simulink subsystem "request_buffer"  (R2021b)
settings: Solver=VariableStepAuto  StartTime=0.0  StopTime=10.0  RelTol=1e-3
undefined symbols (not defined in the file): id_bitwidth, req_mem_size, ts_bitwidth
libraries: hdlsllib x8, simulink x1
settings Model: Creator=torha  LastModifiedBy=torha
settings SolverCC: AlgebraicLoopSolver=TrustRegion
settings DebuggingCC: SFMachineParentedDataDiag=warning

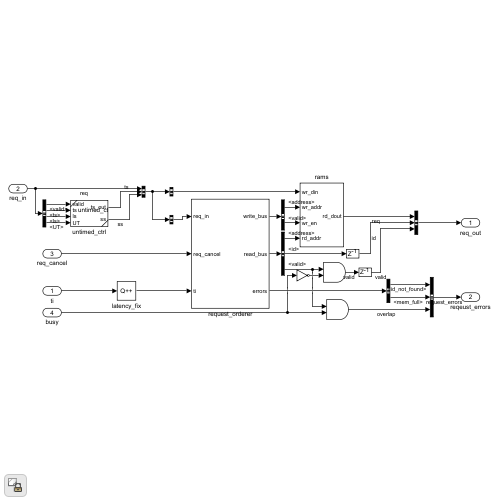
[thumbnail: Simulink's stored preview of the top-level diagram]
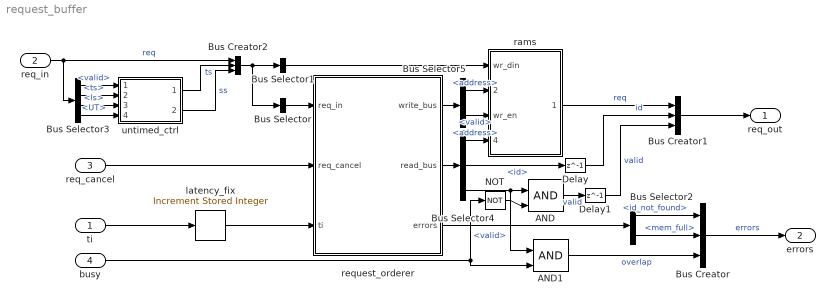
== system request_buffer ==
  ti : Inport
  req_in : Inport  Port=2
  req_cancel : Inport  Port=3
  busy : Inport  Port=4
  AND : Logic  IconShape=distinctive  AllPortsSameDT=off  OutDataTypeStr=boolean
  AND1 : Logic  IconShape=distinctive  AllPortsSameDT=off  OutDataTypeStr=boolean
  Bus Creator : BusCreator  Inputs=3
  Bus Creator1 : BusCreator  Inputs=3
  Bus Creator2 : BusCreator  Inputs=3
  Bus Selector : BusSelector  OutputSignals=req.id,req.valid,ts  OutputAsBus=on
  Bus Selector1 : BusSelector  OutputSignals=req.UC,req.SEND,req.fn,req.filter_address,req.dist_address,ss  OutputAsBus=on
  Bus Selector2 : BusSelector  OutputSignals=signal2.id_not_found,signal2.mem_full
  Bus Selector3 : BusSelector  OutputSignals=valid,ts,ls,UT
  Bus Selector4 : BusSelector  OutputSignals=address,id,valid
  Bus Selector5 : BusSelector  OutputSignals=address,valid
  Delay : Delay  DelayLength=1
  Delay1 : Delay  DelayLength=1
  NOT : Logic  Operator=NOT  IconShape=distinctive  AllPortsSameDT=off  OutDataTypeStr=boolean
  latency_fix : simulink/Additional Math & Discrete/Additional Math: Increment - Decrement/Increment Stored Integer
  rams : Subsystem
  request_orderer : Subsystem
  untimed_ctrl : Subsystem  ReferencedSubsystem=untimed_ctrl
  req_out : Outport
  errors : Outport  Port=2
  wires:
  Bus Selector/1 -> request_orderer/1(req_in)
  busy/1 -> AND1/2, NOT/1
  Bus Creator/1 -> errors/1  "errors"
  AND1/1 -> Bus Creator/3  "overlap"
  req_in/1 -> Bus Creator2/1, Bus Selector3/1  "req"
  NOT/1 -> AND/2
  Bus Selector1/1 -> rams/1(wr_din)
  req_cancel/1 -> request_orderer/2(req_cancel)
  rams/1(rd_dout) -> Bus Creator1/1  "req"
  Bus Selector2/2 -> Bus Creator/2  "<mem_full>"
  Bus Selector2/1 -> Bus Creator/1  "<id_not_found>"
  Bus Creator1/1 -> req_out/1
  Delay/1 -> Bus Creator1/2  "id"
  AND/1 -> Delay1/1  "valid"
  untimed_ctrl/1 -> Bus Creator2/2  "ts"
  Bus Creator2/1 -> Bus Selector1/1, Bus Selector/1
  Bus Selector3/3 -> untimed_ctrl/3  "<ls>"
  Bus Selector3/2 -> untimed_ctrl/2  "<ts>"
  Bus Selector3/4 -> untimed_ctrl/4  "<UT>"
  Bus Selector3/1 -> untimed_ctrl/1  "<valid>"
  untimed_ctrl/2 -> Bus Creator2/3  "ss"
  ti/1 -> latency_fix/1
  Delay1/1 -> Bus Creator1/3  "valid"
  latency_fix/1 -> request_orderer/3(ti)
  request_orderer/3(errors) -> Bus Selector2/1
  request_orderer/2(read_bus) -> Bus Selector4/1
  Bus Selector4/1 -> rams/4(rd_addr)  "<address>"
  Bus Selector5/1 -> rams/2(wr_addr)  "<address>"
  request_orderer/1(write_bus) -> Bus Selector5/1
  Bus Selector5/2 -> rams/3(wr_en)  "<valid>"
  Bus Selector4/3 -> AND/1, AND1/1  "<valid>"
  Bus Selector4/2 -> Delay/1  "<id>"

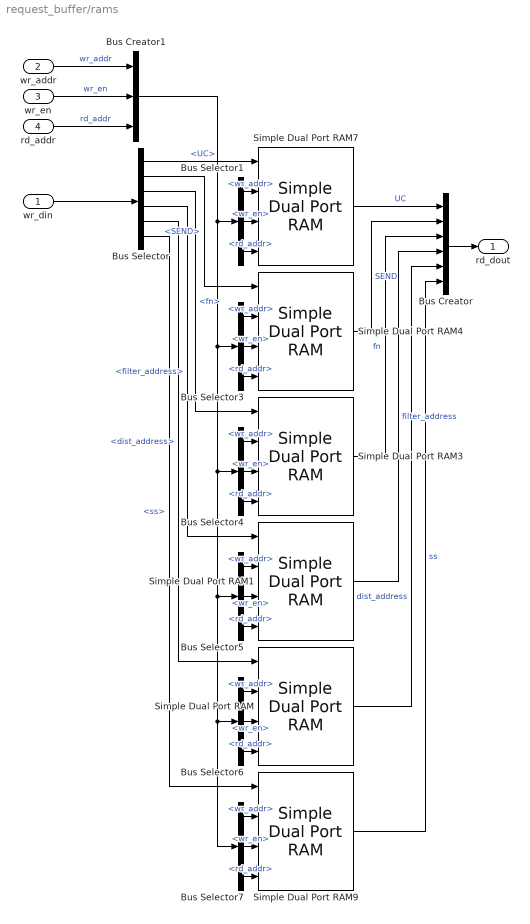
== system request_buffer/rams ==
  wr_din : Inport
  wr_addr : Inport  Port=2
  wr_en : Inport  Port=3
  rd_addr : Inport  Port=4
  Bus Creator : BusCreator  Inputs=6
  Bus Creator1 : BusCreator  Inputs=3
  Bus Selector : BusSelector  OutputSignals=UC,SEND,fn,filter_address,dist_address,ss
  Bus Selector{1,3..7} (6 alike) : BusSelector  OutputSignals=wr_addr,wr_en,rd_addr
  Simple Dual Port RAM{,1,3..4,7,9} (6 alike) : hdlsllib/HDL RAMs/Simple Dual Port RAM  ram_size=log2(req_mem_size)
      settings: SourceProductBaseCode=SL
  rd_dout : Outport
  wires:
  Bus Selector5/3 -> Simple Dual Port RAM1/4  "<rd_addr>"
  Bus Selector5/2 -> Simple Dual Port RAM1/3  "<wr_en>"
  Bus Selector5/1 -> Simple Dual Port RAM1/2  "<wr_addr>"
  Bus Selector4/3 -> Simple Dual Port RAM3/4  "<rd_addr>"
  Bus Selector4/2 -> Simple Dual Port RAM3/3  "<wr_en>"
  Bus Selector4/1 -> Simple Dual Port RAM3/2  "<wr_addr>"
  Bus Creator1/1 -> Bus Selector1/1, Bus Selector7/1, Bus Selector6/1, Bus Selector5/1, Bus Selector4/1, Bus Selector3/1
  Bus Selector6/1 -> Simple Dual Port RAM/2  "<wr_addr>"
  Bus Selector6/2 -> Simple Dual Port RAM/3  "<wr_en>"
  Bus Selector6/3 -> Simple Dual Port RAM/4  "<rd_addr>"
  Bus Selector7/1 -> Simple Dual Port RAM9/2  "<wr_addr>"
  Bus Selector7/2 -> Simple Dual Port RAM9/3  "<wr_en>"
  Bus Selector7/3 -> Simple Dual Port RAM9/4  "<rd_addr>"
  Bus Selector3/3 -> Simple Dual Port RAM4/4  "<rd_addr>"
  Bus Selector3/2 -> Simple Dual Port RAM4/3  "<wr_en>"
  Bus Selector3/1 -> Simple Dual Port RAM4/2  "<wr_addr>"
  Bus Selector1/3 -> Simple Dual Port RAM7/4  "<rd_addr>"
  Bus Selector1/2 -> Simple Dual Port RAM7/3  "<wr_en>"
  Bus Selector1/1 -> Simple Dual Port RAM7/2  "<wr_addr>"
  rd_addr/1 -> Bus Creator1/3  "rd_addr"
  wr_en/1 -> Bus Creator1/2  "wr_en"
  Simple Dual Port RAM9/1 -> Bus Creator/6  "ss"
  Simple Dual Port RAM/1 -> Bus Creator/5  "dist_address"
  Simple Dual Port RAM1/1 -> Bus Creator/4  "filter_address"
  Simple Dual Port RAM3/1 -> Bus Creator/3  "fn"
  Simple Dual Port RAM4/1 -> Bus Creator/2  "SEND"
  Simple Dual Port RAM7/1 -> Bus Creator/1  "UC"
  Bus Creator/1 -> rd_dout/1
  wr_addr/1 -> Bus Creator1/1  "wr_addr"
  wr_din/1 -> Bus Selector/1
  Bus Selector/6 -> Simple Dual Port RAM9/1  "<ss>"
  Bus Selector/5 -> Simple Dual Port RAM/1  "<dist_address>"
  Bus Selector/4 -> Simple Dual Port RAM1/1  "<filter_address>"
  Bus Selector/3 -> Simple Dual Port RAM3/1  "<fn>"
  Bus Selector/2 -> Simple Dual Port RAM4/1  "<SEND>"
  Bus Selector/1 -> Simple Dual Port RAM7/1  "<UC>"

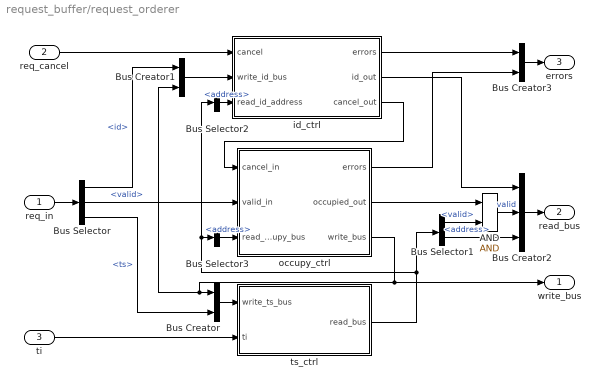
== system request_buffer/request_orderer ==
  req_in : Inport
  req_cancel : Inport  Port=2
  ti : Inport  Port=3
  AND : Logic  IconShape=distinctive  AllPortsSameDT=off  OutDataTypeStr=boolean
  Bus Creator : BusCreator  Inputs=2
  Bus Creator1 : BusCreator  Inputs=2
  Bus Creator2 : BusCreator  Inputs=3
  Bus Creator3 : BusCreator  Inputs=2
  Bus Selector : BusSelector  OutputSignals=id,valid,ts
  Bus Selector1 : BusSelector  OutputSignals=valid,address
  Bus Selector2 : BusSelector  OutputSignals=address
  Bus Selector3 : BusSelector  OutputSignals=address
  id_ctrl : Subsystem
  occupy_ctrl : Subsystem
  ts_ctrl : Subsystem
  write_bus : Outport
  read_bus : Outport  Port=2
  errors : Outport  Port=3
  wires:
  Bus Selector3/1 -> occupy_ctrl/3(read_occupy_bus)  "<address>"
  Bus Creator3/1 -> errors/1
  id_ctrl/1("errors ") -> Bus Creator3/1
  req_cancel/1 -> id_ctrl/1(cancel)
  Bus Selector2/1 -> id_ctrl/3(read_id_address)  "<address>"
  Bus Selector1/2 -> Bus Creator2/3  "<address>"
  Bus Selector1/1 -> AND/2  "<valid>"
  AND/1 -> Bus Creator2/2  "valid"
  occupy_ctrl/1(errors) -> Bus Creator3/2
  id_ctrl/3(cancel_out) -> occupy_ctrl/1(cancel_in)
  id_ctrl/2(id_out) -> Bus Creator2/1
  Bus Creator2/1 -> read_bus/1
  occupy_ctrl/2(occupied_out) -> AND/1
  ts_ctrl/1(read_bus) -> Bus Selector1/1, Bus Selector2/1, Bus Selector3/1
  Bus Creator1/1 -> id_ctrl/2(write_id_bus)
  Bus Creator/1 -> ts_ctrl/1(write_ts_bus)
  occupy_ctrl/3(write_bus) -> write_bus/1, Bus Creator/1, Bus Creator1/2
  Bus Selector/1 -> Bus Creator1/1  "<id>"
  Bus Selector/2 -> occupy_ctrl/2(valid_in)  "<valid>"
  Bus Selector/3 -> Bus Creator/2  "<ts>"
  ti/1 -> ts_ctrl/2(ti)
  req_in/1 -> Bus Selector/1

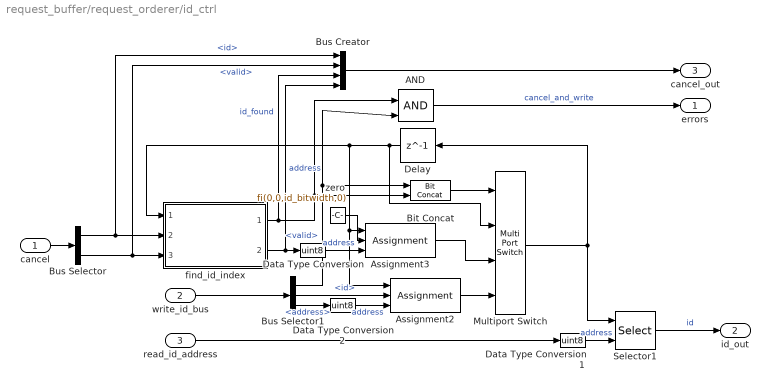
== system request_buffer/request_orderer/id_ctrl ==
  cancel : Inport
  write_id_bus : Inport  Port=2
  read_id_address : Inport  Port=3
  AND : Logic  IconShape=distinctive  AllPortsSameDT=off  OutDataTypeStr=boolean
  Assignment2 : Assignment  IndexMode=Zero-based  IndexOptions=Index vector (port)  Indices=1  OutputSizes=1
  Assignment3 : Assignment  IndexMode=Zero-based  IndexOptions=Index vector (port)  Indices=1  OutputSizes=1
  Bit Concat : hdlsllib/Logic and Bit Operations/Bit Concat  numInputs=2
  Bus Creator : BusCreator  Inputs=4
  Bus Selector : BusSelector  OutputSignals=id,valid
  Bus Selector1 : BusSelector  OutputSignals=available.valid,id,available.address
  Data Type Conversion : DataTypeConversion  OutDataTypeStr=uint8
  Data Type Conversion1 : DataTypeConversion  OutDataTypeStr=uint8
  Data Type Conversion2 : DataTypeConversion  OutDataTypeStr=uint8
  Delay : Delay  DelayLength=1  InitialCondition=fi(zeros(req_mem_size, 1), false, id_bitwidth, 0)
  Multiport Switch : MultiPortSwitch  DataPortOrder=Zero-based contiguous  DataPortIndices={0,1,2}  zeroidx=on
  Selector1 : Selector  IndexMode=Zero-based  InputPortWidth=req_mem_size  IndexOptions=Index vector (port)  Indices=[1 3]  OutputSizes=1
  find_id_index : Subsystem  ReferencedSubsystem=find_id_index
  zero : Constant  Value=fi(0,0,id_bitwidth,0)
  "errors " : Outport
  id_out : Outport  Port=2
  cancel_out : Outport  Port=3
  wires:
  Data Type Conversion2/1 -> Assignment2/3  "address"
  Data Type Conversion1/1 -> Selector1/2  "address"
  Data Type Conversion/1 -> Assignment3/3  "address"
  find_id_index/2 -> Data Type Conversion/1, Bus Creator/4  "address"
  Bus Selector1/1 -> Bit Concat/1, AND/2  "<valid>"
  AND/1 -> "errors "/1  "cancel_and_write"
  Bus Creator/1 -> cancel_out/1
  Bit Concat/1 -> Multiport Switch/1
  find_id_index/1 -> Bit Concat/2, AND/1, Bus Creator/3  "id_found"
  zero/1 -> Assignment3/2
  Assignment3/1 -> Multiport Switch/3
  Bus Selector/2 -> find_id_index/3, Bus Creator/2  "<valid>"
  Bus Selector/1 -> find_id_index/2, Bus Creator/1  "<id>"
  cancel/1 -> Bus Selector/1
  Selector1/1 -> id_out/1  "id"
  read_id_address/1 -> Data Type Conversion1/1
  Delay/1 -> find_id_index/1, Assignment2/1, Assignment3/1, Multiport Switch/2
  Multiport Switch/1 -> Delay/1, Selector1/1
  Bus Selector1/2 -> Assignment2/2  "<id>"
  Bus Selector1/3 -> Data Type Conversion2/1  "<address>"
  Assignment2/1 -> Multiport Switch/4
  write_id_bus/1 -> Bus Selector1/1

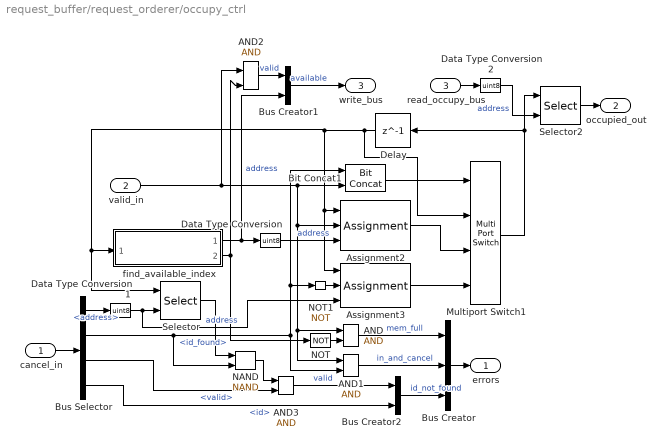
== system request_buffer/request_orderer/occupy_ctrl ==
  cancel_in : Inport
  valid_in : Inport  Port=2
  read_occupy_bus : Inport  Port=3
  AND{,1..3} (4 alike) : Logic  IconShape=distinctive  AllPortsSameDT=off  OutDataTypeStr=boolean
  Assignment2 : Assignment  IndexMode=Zero-based  IndexOptions=Index vector (port)  Indices=1  OutputSizes=1
  Assignment3 : Assignment  IndexMode=Zero-based  IndexOptions=Index vector (port)  Indices=1  OutputSizes=1
  Bit Concat1 : hdlsllib/Logic and Bit Operations/Bit Concat  numInputs=2
  Bus Creator : BusCreator  Inputs=3
  Bus Creator1 : BusCreator  Inputs=2
  Bus Creator2 : BusCreator  Inputs=2
  Bus Selector : BusSelector  OutputSignals=address,id_found,valid,id
  Data Type Conversion : DataTypeConversion  OutDataTypeStr=uint8
  Data Type Conversion1 : DataTypeConversion  OutDataTypeStr=uint8
  Data Type Conversion2 : DataTypeConversion  OutDataTypeStr=uint8
  Delay : Delay  DelayLength=1  InitialCondition=false(req_mem_size, 1)
  Multiport Switch1 : MultiPortSwitch  DataPortOrder=Zero-based contiguous  DataPortIndices={0,1,2}  zeroidx=on
  NAND : Logic  Operator=NAND  IconShape=distinctive  AllPortsSameDT=off  OutDataTypeStr=boolean
  NOT : Logic  Operator=NOT  IconShape=distinctive  AllPortsSameDT=off  OutDataTypeStr=boolean
  NOT1 : Logic  Operator=NOT  IconShape=distinctive  AllPortsSameDT=off  OutDataTypeStr=boolean
  Selector : Selector  IndexMode=Zero-based  IndexOptions=Index vector (port)  Indices=[1 3]  OutputSizes=1
  Selector2 : Selector  IndexMode=Zero-based  IndexOptions=Index vector (port)  Indices=[1 3]  OutputSizes=1
  find_available_index : Subsystem  ReferencedSubsystem=bit64_binary_index_search
  errors : Outport
  occupied_out : Outport  Port=2
  write_bus : Outport  Port=3
  wires:
  NAND/1 -> AND3/1
  Bus Selector/3 -> AND3/2  "<valid>"
  Bus Creator2/1 -> Bus Creator/3  "id_not_found"
  Bus Selector/4 -> Bus Creator2/2  "<id>"
  Data Type Conversion1/1 -> Selector/2, Assignment3/3  "address"
  read_occupy_bus/1 -> Data Type Conversion2/1
  Data Type Conversion2/1 -> Selector2/2  "address"
  Data Type Conversion/1 -> Assignment2/3  "address"
  find_available_index/1 -> Bus Creator1/2, Data Type Conversion/1  "address"
  Selector/1 -> NAND/1
  AND3/1 -> Bus Creator2/1  "valid"
  Bus Creator1/1 -> write_bus/1  "available"
  AND2/1 -> Bus Creator1/1  "valid"
  Bus Creator/1 -> errors/1
  AND1/1 -> Bus Creator/2  "in_and_cancel"
  NOT1/1 -> Assignment3/2
  Bus Selector/1 -> Data Type Conversion1/1  "<address>"
  Bus Selector/2 -> NAND/2, Bit Concat1/1, NOT1/1, AND1/2  "<id_found>"
  AND/1 -> Bus Creator/1  "mem_full"
  NOT/1 -> AND/2
  find_available_index/2 -> NOT/1, AND2/2
  valid_in/1 -> Bit Concat1/2, Assignment2/2, AND/1, AND1/1, AND2/1
  cancel_in/1 -> Bus Selector/1
  Bit Concat1/1 -> Multiport Switch1/1
  Assignment3/1 -> Multiport Switch1/4
  Delay/1 -> find_available_index/1, Selector/1, Assignment2/1, Assignment3/1, Multiport Switch1/2
  Assignment2/1 -> Multiport Switch1/3
  Multiport Switch1/1 -> Selector2/1, Delay/1
  Selector2/1 -> occupied_out/1

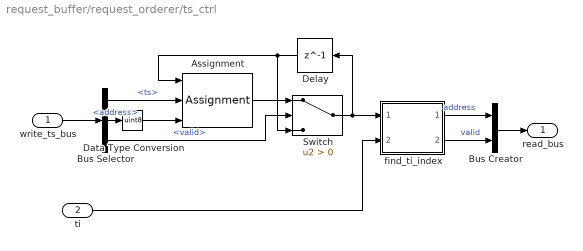
== system request_buffer/request_orderer/ts_ctrl ==
  write_ts_bus : Inport
  ti : Inport  Port=2
  Assignment : Assignment  IndexMode=Zero-based  DiagnosticForDimensions=Warning  IndexOptions=Index vector (port)  Indices=1  OutputSizes=1
  Bus Creator : BusCreator  Inputs=2
  Bus Selector : BusSelector  OutputSignals=ts,available.address,available.valid
  Data Type Conversion : DataTypeConversion  OutDataTypeStr=uint8
  Delay : Delay  DelayLength=1  InitialCondition=fi(zeros(req_mem_size,1),0,ts_bitwidth,0)
  Switch : Switch  Criteria=u2 > Threshold
  find_ti_index : Subsystem  ReferencedSubsystem=find_ti_index
  read_bus : Outport
  wires:
  Data Type Conversion/1 -> Assignment/3
  Bus Creator/1 -> read_bus/1
  write_ts_bus/1 -> Bus Selector/1
  Switch/1 -> find_ti_index/1, Delay/1
  Delay/1 -> Assignment/1, Switch/3
  Assignment/1 -> Switch/1
  Bus Selector/3 -> Switch/2  "<valid>"
  Bus Selector/2 -> Data Type Conversion/1  "<address>"
  Bus Selector/1 -> Assignment/2  "<ts>"
  find_ti_index/1 -> Bus Creator/1  "address"
  find_ti_index/2 -> Bus Creator/2  "valid"
  ti/1 -> find_ti_index/2
